simulink model "gain_selection_ex"  (R2022a)
settings: Solver=VariableStepAuto  StartTime=0.0  StopTime=tspan  RelTol=1e-3  EnableMultiTasking=on
values from neighbouring files (symbols this model uses):
  J = diag([20 30 40])    [gain_selection_ex_init.m]
  Kd = J*eye(3)*2*zeta*wn    [gain_selection_ex_init.m]
  Kp = 2*J*eye(3)*wn^2    [gain_selection_ex_init.m]
  q_b_ECI_0 = [epsilon_b_ECI_0; sqrt(1-norm(epsilon_b_ECI_0)^2)]    [gain_selection_ex_init.m]
  q_C = [epsilon_C; sqrt(1-norm(epsilon_C)^2)]    [gain_selection_ex_init.m]
  w_0 = [.1; -.1; .2]    [gain_selection_ex_init.m]
settings Model: Creator=emehiel  LastModifiedBy=emehiel
settings SolverCC: AlgebraicLoopSolver=TrustRegion
settings DataIOCC: SaveFormat=Array  ReturnWorkspaceOutputs=off
settings OptimizationCC: LifeSpan=inf
settings DebuggingCC: UnconnectedInputMsg=warning  UnconnectedOutputMsg=warning  UnconnectedLineMsg=warning  AllowSymbolicDim=off  SFUnexpectedBacktrackingDiag=warning  SFNoUnconditionalDefaultTransitionDiag=warning  SFExecutionAtInitializationDiag=none  SFMachineParentedDataDiag=warning  ArithmeticOperatorsInVariantConditions=warning
settings ModelReferenceCC: PropagateSignalLabelsOutOfModel=off
settings SFSimCC: SimUseLocalCustomCode=off  CustomCodeUndefinedFunction=UseInterfaceOnly
settings RTWCC: RTWUseLocalCustomCode=off
settings CodeAppCC: StateflowObjectComments=on
settings GRTTargetCC: TargetLangStandard=C89/C90 (ANSI)
settings ConfigComp: CovMetricSettings=dw  CovSaveCumulativeToWorkspaceVar=on  CovSaveSingleToWorkspaceVar=on  CovExternalEMLEnable=off

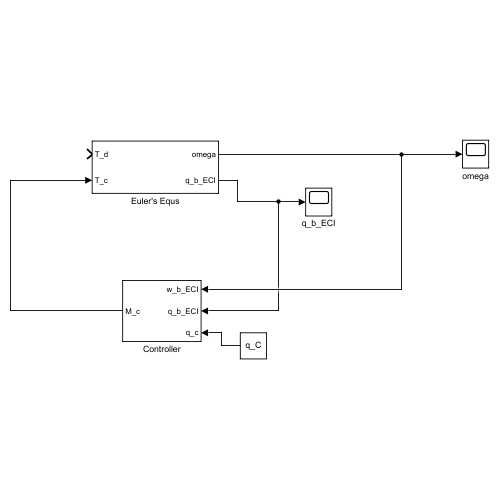
[thumbnail: Simulink's stored preview of the top-level diagram]
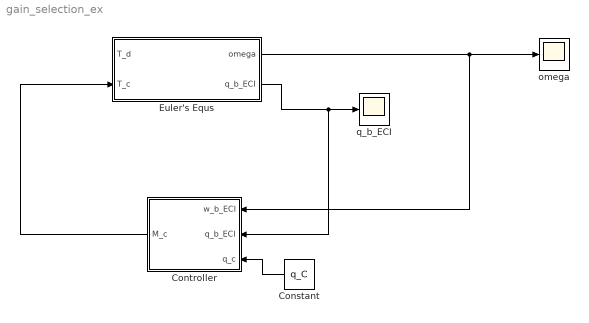
== system gain_selection_ex ==
  Constant : Constant  Value=q_C
  Controller : Subsystem
  Euler's Equs : Subsystem
  omega : Scope
  q_b_ECI : Scope
  wires:
  Euler's Equs/1(omega) -> Controller/1(w_b_ECI), omega/1
  Euler's Equs/2(q_b_ECI) -> Controller/2(q_b_ECI), q_b_ECI/1
  Controller/1(M_c) -> Euler's Equs/2(T_c)
  Constant/1 -> Controller/3(q_c)

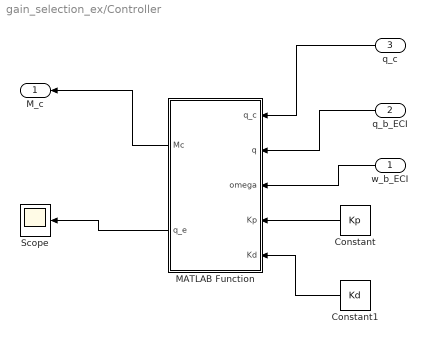
== system gain_selection_ex/Controller ==
  w_b_ECI : Inport  PortDimensions=[3 1]
  q_b_ECI : Inport  Port=2  PortDimensions=[4 1]
  q_c : Inport  Port=3  PortDimensions=[4 1]
  Constant : Constant  Value=Kp
  Constant1 : Constant  Value=Kd
  MATLAB Function : MATLAB Function  TreatAsAtomicUnit=on
  Scope : Scope
  M_c : Outport  PortDimensions=[3 1]  VectorParamsAs1DForOutWhenUnconnected=off
  wires:
  MATLAB Function/1(Mc) -> M_c/1
  q_c/1 -> MATLAB Function/1(q_c)
  q_b_ECI/1 -> MATLAB Function/2(q)
  w_b_ECI/1 -> MATLAB Function/3(omega)
  Constant/1 -> MATLAB Function/4(Kp)
  Constant1/1 -> MATLAB Function/5(Kd)
  MATLAB Function/2(q_e) -> Scope/1

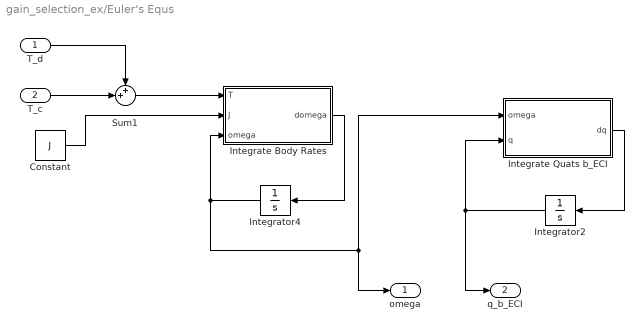
== system gain_selection_ex/Euler's Equs ==
  T_d : Inport
  T_c : Inport  Port=2
  Constant : Constant  Value=J
  Integrate Body Rates : MATLAB Function  TreatAsAtomicUnit=on
  Integrate Quats b_ECI : MATLAB Function  TreatAsAtomicUnit=on
  Integrator2 : Integrator  InitialCondition=q_b_ECI_0
  Integrator4 : Integrator  InitialCondition=w_0
  Sum1 : Sum  Inputs=++|
  omega : Outport
  q_b_ECI : Outport  Port=2  PortDimensions=[4 1]
  wires:
  Integrate Body Rates/1(domega) -> Integrator4/1
  Constant/1 -> Integrate Body Rates/2(J)
  Integrate Quats b_ECI/1(dq) -> Integrator2/1
  Integrator2/1 -> q_b_ECI/1, Integrate Quats b_ECI/2(q)
  Integrator4/1 -> Integrate Quats b_ECI/1(omega), omega/1, Integrate Body Rates/3(omega)
  T_c/1 -> Sum1/2
  Sum1/1 -> Integrate Body Rates/1(T)
  T_d/1 -> Sum1/1

== matlab function gain_selection_ex/Euler's Equs/Integrate Body Rates ==
  data: T input; J input; omega input; domega output
function domega = dynamics(T, J, omega)
%#codegen

domega = J\(T - cross(omega, J*omega));

== matlab function gain_selection_ex/Euler's Equs/Integrate Quats b_ECI ==
  data: omega input; q input; dq output
function dq = kinematics(omega, q)
%#codegen

% unpack quaternion

epsilon = q(1:3,1);
eta = q(4,1);

depsilon = 1/2*(eta*eye(3) + vect2cross(epsilon))*omega;
deta = -1/2*epsilon'*omega;

dq = [depsilon; deta];

== matlab function gain_selection_ex/Controller/MATLAB Function ==
  data: q_c input; Mc output; q input; omega input; Kp input; Kd input; q_e output
function [Mc,q_e]  = control_law(q_c, q, omega, Kp, Kd)
%#codegen

%q_e = quatMult(quatConjugate(q_c), q);
q_e = quatMult(q, quatConjugate(q_c));
Mc = -Kp*q_e(1:3,1) - Kd*omega;
